simulink model "PMSM_mathmodel"  (R2018a)
settings: Solver=VariableStepAuto  StartTime=0.0  StopTime=2  RelTol=1e-3
libraries: nesl_utility x14, fl_lib x14, simulink x2, elec_lib x1
settings Model: Creator=Arpan  LastModifiedBy=Arpan

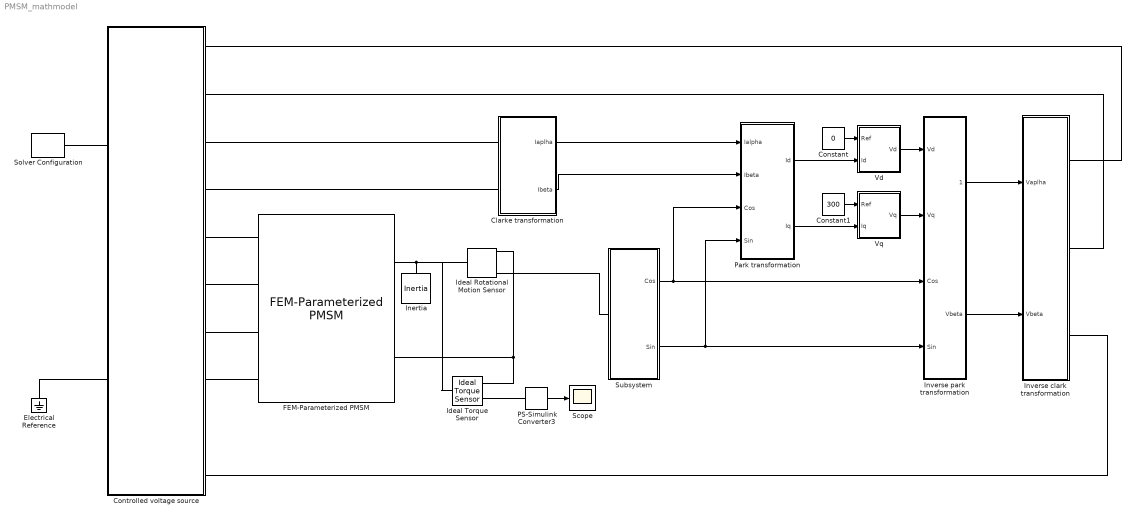
== system PMSM_mathmodel ==
  Clarke transformation : Subsystem
  Constant : Constant  Value=0
  Constant1 : Constant  Value=300
  Controlled voltage source : Subsystem
  Electrical Reference : fl_lib/Electrical/Electrical Elements/Electrical Reference
  FEM-Parameterized PMSM : elec_lib/Actuators & Drivers/Rotational Actuators/FEM-Parameterized PMSM  parameterization=2  iVec=[-2, 0, 2] A  xVec=[0, 20, 40, 60] deg  dfluxdiMatrix=0.0002 * ones(3, 4) Wb/A  dfluxdxMatrix=[0, -.16, .16, 0; 0, -.16, .16, 0; 0, -.16, .16, 0] Wb/rad  calculate_torque_matrix=1  TorqueMatrix=zeros(3, 3, 3, 4) N*m  idVec1=[-200, 0, 200] A  iqVec1=[-200, 0, 200] A  LdMatrix=0.0002 * ones(3, 3) H  LqMatrix=0.0002 * ones(3, 3) H  PmMatrix=0.1 * ones(3, 3) Wb  N=10  interp_method=simscape.enum.interpolation.linear  Rs=0.013 Ohm  Ms=0.00002 H  losses_oc=[0, 0, 0] W  losses_sc=[0, 0, 0] W  f_losses=60 Hz  Isc_losses=95 A  Inertia=0.1 kg*m^2  lam=0 N*m/(rad/s)  i_d_specify=on  i_d_priority=None  i_d=0.0085 A  i_d_nominal_specify=off  i_d_nominal_unit=A  i_d_nominal_value=1  i_q_specify=on  i_q_priority=None  i_q=0.0085 A  i_q_nominal_specify=off  i_q_nominal_unit=A  i_q_nominal_value=1  torque_specify=off  torque_priority=None  torque=0 N*m  torque_nominal_specify=off  torque_nominal_unit=N*m  torque_nominal_value=1  angular_velocity_specify=off  angular_velocity_priority=High  angular_velocity=0 rpm  angular_velocity_nominal_specify=off  angular_velocity_nominal_unit=rpm  angular_velocity_nominal_value=1  angular_position_specify=off  angular_position_priority=High  angular_position=0 deg  angular_position_nominal_specify=off  angular_position_nominal_unit=deg  angular_position_nominal_value=1  Tmeas=298.15 K  alpha=3.93e-3 1/K  alpha_flux=-0.001 1/K  stator_thermal_mass=100 J/K  stator_initial_temperatures=[298.15, 298.15, 298.15] K  rotor_thermal_mass=200 J/K  rotor_initial_temperature=298.15 K  Rm_percent_rotor=90  Rd_percent_rotor=30  idVec=[-200, 0, 200] A  iqVec=[-200, 0, 200] A  dfluxAdiaMatrix3D=zeros(3, 3, 4) Wb/A  dfluxAdibMatrix3D=zeros(3, 3, 4) Wb/A  dfluxAdicMatrix3D=zeros(3, 3, 4) Wb/A  dfluxAdxMatrix3D=zeros(3, 3, 4) Wb/rad  TorqueMatrix3D=zeros(3, 3, 4) N*m  iaVec=[-200, 0, 200] A  ibVec=[-200, 0, 200] A  icVec=[-200, 0, 200] A  dfluxAdiaMatrix=zeros(3, 3, 3, 4) Wb/A  dfluxAdibMatrix=zeros(3, 3, 3, 4) Wb/A  dfluxAdicMatrix=zeros(3, 3, 3, 4) Wb/A  dfluxAdxMatrix=zeros(3, 3, 3, 4) Wb/rad  winding_type_dq0=1  nPolePairs=4  parks_type=1  idVec2=[-200, 0, 200] A  iqVec2=[-200, 0, 200] A  xVec2=[0, 10, 20, 30] deg  fluxD_dq0=zeros(3, 3, 4) Wb  fluxQ_dq0=zeros(3, 3, 4) Wb  Torque_dq0=zeros(3, 3, 4) N*m
      settings: SourceProductName=Simscape Electronics  SourceProductBaseCode=SN
  Ideal Rotational Motion Sensor : fl_lib/Mechanical/Mechanical Sensors/Ideal Rotational Motion Sensor  offset=48 deg
  Ideal Torque Sensor : fl_lib/Mechanical/Mechanical Sensors/Ideal Torque Sensor
  Inertia : fl_lib/Mechanical/Rotational Elements/Inertia  inertia=0.01 kg*m^2  w_specify=off  w_priority=High  w=0 rad/s  w_nominal_specify=off  w_nominal_unit=rad/s  w_nominal_value=1  t_specify=off  t_priority=None  t=0 N*m  t_nominal_specify=off  t_nominal_unit=N*m  t_nominal_value=1
  Inverse clark transformation : Subsystem
  Inverse park transformation : Subsystem
  PS-Simulink Converter3 : nesl_utility/PS-Simulink Converter  PhysicalDomain=network_engine_domain  SubClassName=ps_output  LeftPortType=input  RightPortType=output  PseudoPeriodic=off  Frequencies=[]  Unit=1  AffineConversion=off
  Park transformation : Subsystem
  Scope : Scope
  Solver Configuration : nesl_utility/Solver Configuration  PhysicalDomain=network_engine_domain  SubClassName=solver  LeftPortType=input  RightPortType=generic  Tones=[]  Harmonics=[]  SimulateNoise=off  Profile=off  UseLocalSampling=off  EnableSwitchedLinearOptims=on  FrequencyDomain=off  UseCCode=off  RelTol=0.001  AbsTol=1e-06  MinStep=1e-09  ToWorkspace=off  RevertToSquareIcSolve=off  NumHomotopyIterations=100  PhasorMode=off  PhasorModeNumHarmonics=1  DoDC=off  ResidualTolerance=1e-09  UseLocalSolver=off  LocalSolverChoice=NE_BACKWARD_EULER_ADVANCER  LocalSolverSampleTime=0.001  DoFixedCost=off  MaxNonlinIter=3  MaxModeIter=2  LinearAlgebra=Sparse  EquationFormulation=NE_TIME_EF  DelaysMemoryBudget=1024  AutomaticFiltering=on  FilteringTimeConstant=0.001
  Subsystem : Subsystem
  Vd : Subsystem
  Vq : Subsystem
  wires:
  PS-Simulink Converter3/1 -> Scope/1
  Constant/1 -> Vd/1(Ref)
  Constant1/1 -> Vq/1(Ref)
  Clarke transformation/1(Iaplha) -> Park transformation/1(Ialpha)
  Clarke transformation/2(Ibeta) -> Park transformation/2(Ibeta)
  Park transformation/1(Id) -> Vd/2(Id)
  Park transformation/2(Iq) -> Vq/2(Iq)
  Vd/1(Vd) -> Inverse park transformation/1(Vd)
  Vq/1(Vq) -> Inverse park transformation/2(Vq)
  Inverse park transformation/1(Valpha) -> Inverse clark transformation/1(Vaplha)
  Inverse park transformation/2(Vbeta) -> Inverse clark transformation/2(Vbeta)
  Subsystem/1(Cos) -> Inverse park transformation/3(Cos), Park transformation/3(Cos)
  Subsystem/2(Sin) -> Inverse park transformation/4(Sin), Park transformation/4(Sin)
  connections:
  FEM-Parameterized PMSM/RConn1 -- Ideal Torque Sensor/LConn1 -- Ideal Rotational Motion Sensor/LConn1 -- Inertia/LConn1
  FEM-Parameterized PMSM/RConn2 -- Ideal Rotational Motion Sensor/RConn1 -- Ideal Torque Sensor/RConn1
  PS-Simulink Converter3/LConn1 -- Ideal Torque Sensor/RConn2
  Solver Configuration/RConn1 -- Controlled voltage source/LConn1
  Controlled voltage source/RConn3 -- Clarke transformation/LConn1
  Controlled voltage source/RConn4 -- Clarke transformation/LConn2
  Controlled voltage source/RConn5 -- FEM-Parameterized PMSM/LConn1
  Controlled voltage source/RConn6 -- FEM-Parameterized PMSM/LConn2
  Controlled voltage source/RConn7 -- FEM-Parameterized PMSM/LConn3
  Controlled voltage source/RConn8 -- FEM-Parameterized PMSM/LConn4
  Controlled voltage source/LConn2 -- Electrical Reference/LConn1
  Inverse clark transformation/RConn1 -- Controlled voltage source/RConn1
  Inverse clark transformation/RConn2 -- Controlled voltage source/RConn2
  Inverse clark transformation/RConn3 -- Controlled voltage source/RConn10
  Subsystem/LConn1 -- Ideal Rotational Motion Sensor/RConn3

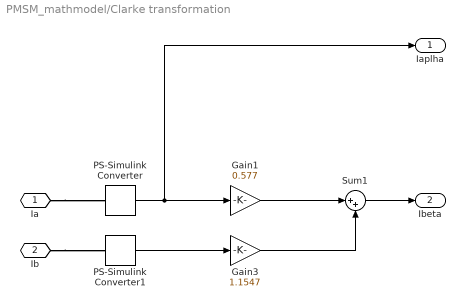
== system PMSM_mathmodel/Clarke transformation ==
  Gain1 : Gain  Gain=0.577
  Gain3 : Gain  Gain=1.1547
  PS-Simulink Converter : nesl_utility/PS-Simulink Converter  PhysicalDomain=network_engine_domain  SubClassName=ps_output  LeftPortType=input  RightPortType=output  PseudoPeriodic=off  Frequencies=[]  Unit=1  AffineConversion=off
  PS-Simulink Converter1 : nesl_utility/PS-Simulink Converter  PhysicalDomain=network_engine_domain  SubClassName=ps_output  LeftPortType=input  RightPortType=output  PseudoPeriodic=off  Frequencies=[]  Unit=1  AffineConversion=off
  Sum1 : Sum  Inputs=|++
  Ia : PMIOPort  Side=Left
  Ib : PMIOPort  Port=2  Side=Left
  Iaplha : Outport
  Ibeta : Outport  Port=2
  wires:
  Sum1/1 -> Ibeta/1
  Gain1/1 -> Sum1/1
  PS-Simulink Converter/1 -> Gain1/1, Iaplha/1
  Gain3/1 -> Sum1/2
  PS-Simulink Converter1/1 -> Gain3/1
  connections:
  Ib/RConn1 -- PS-Simulink Converter1/LConn1
  Ia/RConn1 -- PS-Simulink Converter/LConn1

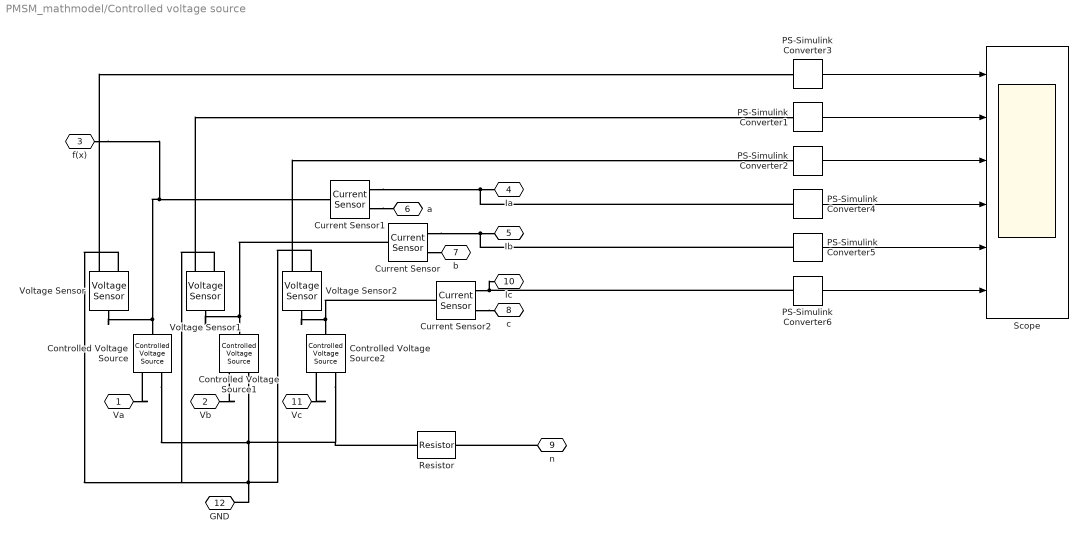
== system PMSM_mathmodel/Controlled voltage source ==
  Controlled Voltage Source : fl_lib/Electrical/Electrical Sources/Controlled Voltage Source
  Controlled Voltage Source1 : fl_lib/Electrical/Electrical Sources/Controlled Voltage Source
  Controlled Voltage Source2 : fl_lib/Electrical/Electrical Sources/Controlled Voltage Source
  Current Sensor : fl_lib/Electrical/Electrical Sensors/Current Sensor
  Current Sensor1 : fl_lib/Electrical/Electrical Sensors/Current Sensor
  Current Sensor2 : fl_lib/Electrical/Electrical Sensors/Current Sensor
  PS-Simulink Converter{1..6} (6 alike) : nesl_utility/PS-Simulink Converter  PhysicalDomain=network_engine_domain  SubClassName=ps_output  LeftPortType=input  RightPortType=output  PseudoPeriodic=off  Frequencies=[]  Unit=1  AffineConversion=off
  Resistor : fl_lib/Electrical/Electrical Elements/Resistor  R=1000 Ohm  i_specify=off  i_priority=None  i=0 A  i_nominal_specify=off  i_nominal_unit=A  i_nominal_value=1  v_specify=off  v_priority=None  v=0 V  v_nominal_specify=off  v_nominal_unit=V  v_nominal_value=1
  Scope : Scope  NumInputPorts=6
  Voltage Sensor : fl_lib/Electrical/Electrical Sensors/Voltage Sensor
  Voltage Sensor1 : fl_lib/Electrical/Electrical Sensors/Voltage Sensor
  Voltage Sensor2 : fl_lib/Electrical/Electrical Sensors/Voltage Sensor
  Va : PMIOPort  Side=Right
  Vb : PMIOPort  Port=2  Side=Right
  f(x) : PMIOPort  Port=3  Side=Left
  Ia : PMIOPort  Port=4  Side=Right
  Ib : PMIOPort  Port=5  Side=Right
  a : PMIOPort  Port=6  Side=Right
  b : PMIOPort  Port=7  Side=Right
  c : PMIOPort  Port=8  Side=Right
  n : PMIOPort  Port=9  Side=Right
  Ic : PMIOPort  Port=10  Side=Right
  Vc : PMIOPort  Port=11  Side=Right
  GND : PMIOPort  Port=12  Side=Left
  wires:
  PS-Simulink Converter3/1 -> Scope/1
  PS-Simulink Converter1/1 -> Scope/2
  PS-Simulink Converter2/1 -> Scope/3
  PS-Simulink Converter4/1 -> Scope/4
  PS-Simulink Converter5/1 -> Scope/5
  PS-Simulink Converter6/1 -> Scope/6
  connections:
  Current Sensor2/RConn1 -- Ic/RConn1 -- PS-Simulink Converter6/LConn1
  Current Sensor/RConn2 -- b/RConn1
  Current Sensor2/RConn2 -- c/RConn1
  Controlled Voltage Source/RConn2 -- Resistor/RConn1 -- Controlled Voltage Source2/RConn2 -- Voltage Sensor1/RConn2 -- Voltage Sensor/RConn2 -- Voltage Sensor2/RConn2 -- GND/RConn1 -- Controlled Voltage Source1/RConn2
  Current Sensor1/RConn1 -- PS-Simulink Converter4/LConn1 -- Ia/RConn1
  Current Sensor1/RConn2 -- a/RConn1
  Va/RConn1 -- Controlled Voltage Source/RConn1
  Vb/RConn1 -- Controlled Voltage Source1/RConn1
  Vc/RConn1 -- Controlled Voltage Source2/RConn1
  Current Sensor/RConn1 -- PS-Simulink Converter5/LConn1 -- Ib/RConn1
  f(x)/RConn1 -- Voltage Sensor/LConn1 -- Controlled Voltage Source/LConn1 -- Current Sensor1/LConn1
  Current Sensor/LConn1 -- Voltage Sensor1/LConn1 -- Controlled Voltage Source1/LConn1
  Current Sensor2/LConn1 -- Voltage Sensor2/LConn1 -- Controlled Voltage Source2/LConn1
  Voltage Sensor/RConn1 -- PS-Simulink Converter3/LConn1
  Voltage Sensor1/RConn1 -- PS-Simulink Converter1/LConn1
  Voltage Sensor2/RConn1 -- PS-Simulink Converter2/LConn1
  n/RConn1 -- Resistor/LConn1

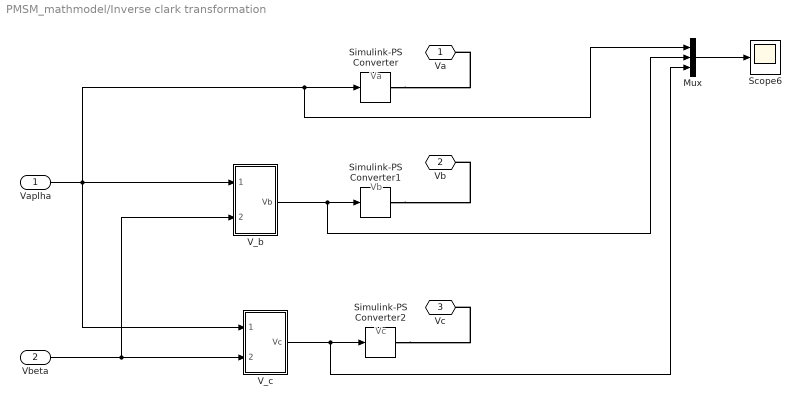
== system PMSM_mathmodel/Inverse clark transformation ==
  note: Vc
  note: Vb
  note: Va
  Vaplha : Inport
  Vbeta : Inport  Port=2
  Mux : Mux  Inputs=3
  Scope6 : Scope
  Simulink-PS Converter : nesl_utility/Simulink-PS Converter  PhysicalDomain=network_engine_domain  SubClassName=ps_input  LeftPortType=input  RightPortType=output  PseudoPeriodic=off  Frequencies=[]  NoiseDistribution=none  NoiseParameters=[]  Unit=1  AffineConversion=off  FilteringAndDerivatives=provide  SimscapeFilterOrder=1  InputFilterTimeConstant=0.001  UdotUserProvided=0
  Simulink-PS Converter1 : nesl_utility/Simulink-PS Converter  PhysicalDomain=network_engine_domain  SubClassName=ps_input  LeftPortType=input  RightPortType=output  PseudoPeriodic=off  Frequencies=[]  NoiseDistribution=none  NoiseParameters=[]  Unit=1  AffineConversion=off  FilteringAndDerivatives=provide  SimscapeFilterOrder=1  InputFilterTimeConstant=0.001  UdotUserProvided=0
  Simulink-PS Converter2 : nesl_utility/Simulink-PS Converter  PhysicalDomain=network_engine_domain  SubClassName=ps_input  LeftPortType=input  RightPortType=output  PseudoPeriodic=off  Frequencies=[]  NoiseDistribution=none  NoiseParameters=[]  Unit=1  AffineConversion=off  FilteringAndDerivatives=provide  SimscapeFilterOrder=1  InputFilterTimeConstant=0.001  UdotUserProvided=0
  V_b : Subsystem
  V_c : Subsystem
  Va : PMIOPort  Side=Right
  Vb : PMIOPort  Port=2  Side=Right
  Vc : PMIOPort  Port=3  Side=Right
  wires:
  Vbeta/1 -> V_c/2(Vbeta), V_b/2(Vbeta)
  Mux/1 -> Scope6/1
  V_c/1(Vc) -> Mux/3, Simulink-PS Converter2/1
  Vaplha/1 -> Mux/1, Simulink-PS Converter/1, V_b/1(Valpha), V_c/1(Valpha)
  V_b/1(Vb) -> Mux/2, Simulink-PS Converter1/1
  connections:
  Simulink-PS Converter1/RConn1 -- Vb/RConn1
  Simulink-PS Converter2/RConn1 -- Vc/RConn1
  Simulink-PS Converter/RConn1 -- Va/RConn1

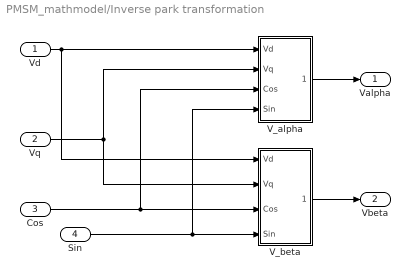
== system PMSM_mathmodel/Inverse park transformation ==
  Vd : Inport
  Vq : Inport  Port=2
  Cos : Inport  Port=3
  Sin : Inport  Port=4
  V_alpha : Subsystem
  V_beta : Subsystem
  Valpha : Outport
  Vbeta : Outport  Port=2
  wires:
  Sin/1 -> V_alpha/4(Sin), V_beta/4(Sin)
  Vd/1 -> V_alpha/1(Vd), V_beta/1(Vd)
  Cos/1 -> V_alpha/3(Cos), V_beta/3(Cos)
  V_beta/1(Vbeta) -> Vbeta/1
  V_alpha/1(Valpha) -> Valpha/1
  Vq/1 -> V_beta/2(Vq), V_alpha/2(Vq)

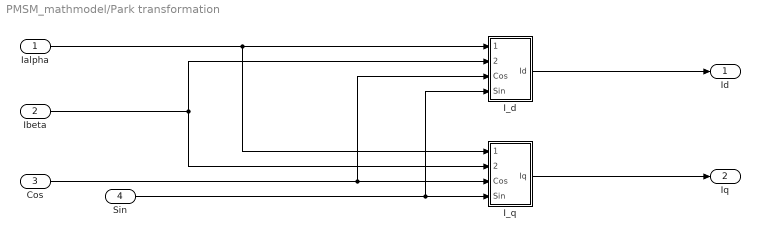
== system PMSM_mathmodel/Park transformation ==
  Ialpha : Inport
  Ibeta : Inport  Port=2
  Cos : Inport  Port=3
  Sin : Inport  Port=4
  I_d : Subsystem
  I_q : Subsystem
  Id : Outport
  Iq : Outport  Port=2
  wires:
  Cos/1 -> I_q/3(Cos), I_d/3(Cos)
  Ialpha/1 -> I_q/1(Ialpha), I_d/1(Iaplha)
  I_q/1(Iq) -> Iq/1
  Ibeta/1 -> I_q/2(Ibeta), I_d/2(Ibeta)
  Sin/1 -> I_d/4(Sin), I_q/4(Sin)
  I_d/1(Id) -> Id/1

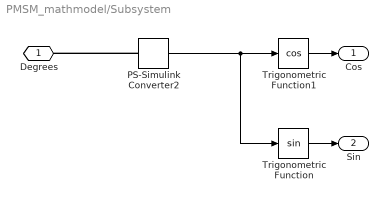
== system PMSM_mathmodel/Subsystem ==
  PS-Simulink Converter2 : nesl_utility/PS-Simulink Converter  PhysicalDomain=network_engine_domain  SubClassName=ps_output  LeftPortType=input  RightPortType=output  PseudoPeriodic=off  Frequencies=[]  Unit=1  AffineConversion=off
  Trigonometric Function : Trigonometry
  Trigonometric Function1 : Trigonometry  Operator=cos
  "Degrees " : PMIOPort  Side=Left
  Cos : Outport
  Sin : Outport  Port=2
  wires:
  PS-Simulink Converter2/1 -> Trigonometric Function/1, Trigonometric Function1/1
  Trigonometric Function1/1 -> Cos/1
  Trigonometric Function/1 -> Sin/1
  connections:
  PS-Simulink Converter2/LConn1 -- "Degrees "/RConn1

== system PMSM_mathmodel/Vd ==
  Ref : Inport
  Id : Inport  Port=2
  PID Controller (2DOF) : simulink/Continuous/PID Controller (2DOF)  Controller=PI  TimeDomain=Continuous-time  SampleTime=-1  IntegratorMethod=Forward Euler  FilterMethod=Forward Euler  Form=Parallel  UseFilter=on  ControllerParametersSource=internal  P=10  I=5  D=0  N=100  b=1  c=1  InitialConditionSource=internal  InitialConditionForIntegrator=0  InitialConditionForFilter=0  ExternalReset=none  LimitOutput=off  UpperSaturationLimit=inf  LowerSaturationLimit=-inf  LinearizeAsGain=on  AntiWindupMode=none  Kb=1  TrackingMode=off  Kt=1  PParamMin=[]  PParamMax=[]  IParamMin=[]  IParamMax=[]  DParamMin=[]  DParamMax=[]  NParamMin=[]  NParamMax=[]  bParamMin=[]  bParamMax=[]  cParamMin=[]  cParamMax=[]  KbParamMin=[]  KbParamMax=[]  KtParamMin=[]  KtParamMax=[]  POutMin=[]  POutMax=[]  IOutMin=[]  IOutMax=[]  DOutMin=[]  DOutMax=[]  NOutMin=[]  NOutMax=[]  bOutMin=[]  bOutMax=[]  cOutMin=[]  cOutMax=[]  KbOutMin=[]  KbOutMax=[]  KtOutMin=[]  KtOutMax=[]  IntegratorOutMin=[]  IntegratorOutMax=[]  FilterOutMin=[]  FilterOutMax=[]  SumOutMin=[]  SumOutMax=[]  Sum1OutMin=[]  Sum1OutMax=[]  Sum2OutMin=[]  Sum2OutMax=[]  Sum3OutMin=[]  Sum3OutMax=[]  SumI1OutMin=[]  SumI1OutMax=[]  SumI2OutMin=[]  SumI2OutMax=[]  SumI3OutMin=[]  SumI3OutMax=[]  SumDOutMin=[]  SumDOutMax=[]  SaturationOutMin=[]  SaturationOutMax=[]  IntegratorContinuousStateAttributes=''  IntegratorStateMustResolveToSignalObject=off  IntegratorRTWStateStorageClass=Auto  FilterContinuousStateAttributes=''  FilterStateMustResolveToSignalObject=off  FilterRTWStateStorageClass=Auto  DifferentiatorICPrevScaledInput=0  DifferentiatorOutMin=[]  DifferentiatorOutMax=[]  FilterDiffOutCoefMin=[]  FilterDiffOutCoefMax=[]  SumDenOutMin=[]  SumDenOutMax=[]  SumNumOutMin=[]  SumNumOutMax=[]  ReciprocalOutMin=[]  ReciprocalOutMax=[]  DivideOutMin=[]  DivideOutMax=[]  TunerSelectOption=Transfer Function Based (PID Tuner App)
  Vd : Outport
  wires:
  PID Controller (2DOF)/1 -> Vd/1
  Ref/1 -> PID Controller (2DOF)/1
  Id/1 -> PID Controller (2DOF)/2

== system PMSM_mathmodel/Vq ==
  Ref : Inport
  Iq : Inport  Port=2
  PID Controller (2DOF)1 : simulink/Continuous/PID Controller (2DOF)  Controller=PI  TimeDomain=Continuous-time  SampleTime=-1  IntegratorMethod=Forward Euler  FilterMethod=Forward Euler  Form=Parallel  UseFilter=on  ControllerParametersSource=internal  P=10  I=5  D=0  N=100  b=1  c=1  InitialConditionSource=internal  InitialConditionForIntegrator=0  InitialConditionForFilter=0  ExternalReset=none  LimitOutput=off  UpperSaturationLimit=inf  LowerSaturationLimit=-inf  LinearizeAsGain=on  AntiWindupMode=none  Kb=1  TrackingMode=off  Kt=1  PParamMin=[]  PParamMax=[]  IParamMin=[]  IParamMax=[]  DParamMin=[]  DParamMax=[]  NParamMin=[]  NParamMax=[]  bParamMin=[]  bParamMax=[]  cParamMin=[]  cParamMax=[]  KbParamMin=[]  KbParamMax=[]  KtParamMin=[]  KtParamMax=[]  POutMin=[]  POutMax=[]  IOutMin=[]  IOutMax=[]  DOutMin=[]  DOutMax=[]  NOutMin=[]  NOutMax=[]  bOutMin=[]  bOutMax=[]  cOutMin=[]  cOutMax=[]  KbOutMin=[]  KbOutMax=[]  KtOutMin=[]  KtOutMax=[]  IntegratorOutMin=[]  IntegratorOutMax=[]  FilterOutMin=[]  FilterOutMax=[]  SumOutMin=[]  SumOutMax=[]  Sum1OutMin=[]  Sum1OutMax=[]  Sum2OutMin=[]  Sum2OutMax=[]  Sum3OutMin=[]  Sum3OutMax=[]  SumI1OutMin=[]  SumI1OutMax=[]  SumI2OutMin=[]  SumI2OutMax=[]  SumI3OutMin=[]  SumI3OutMax=[]  SumDOutMin=[]  SumDOutMax=[]  SaturationOutMin=[]  SaturationOutMax=[]  IntegratorContinuousStateAttributes=''  IntegratorStateMustResolveToSignalObject=off  IntegratorRTWStateStorageClass=Auto  FilterContinuousStateAttributes=''  FilterStateMustResolveToSignalObject=off  FilterRTWStateStorageClass=Auto  DifferentiatorICPrevScaledInput=0  DifferentiatorOutMin=[]  DifferentiatorOutMax=[]  FilterDiffOutCoefMin=[]  FilterDiffOutCoefMax=[]  SumDenOutMin=[]  SumDenOutMax=[]  SumNumOutMin=[]  SumNumOutMax=[]  ReciprocalOutMin=[]  ReciprocalOutMax=[]  DivideOutMin=[]  DivideOutMax=[]  TunerSelectOption=Transfer Function Based (PID Tuner App)
  Vq : Outport
  wires:
  PID Controller (2DOF)1/1 -> Vq/1
  Ref/1 -> PID Controller (2DOF)1/1
  Iq/1 -> PID Controller (2DOF)1/2

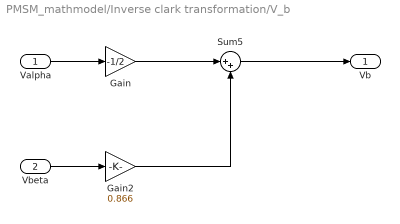
== system PMSM_mathmodel/Inverse clark transformation/V_b ==
  Valpha : Inport
  Vbeta : Inport  Port=2
  Gain : Gain  Gain=-1/2
  Gain2 : Gain  Gain=0.866
  Sum5 : Sum  Inputs=|++
  Vb : Outport
  wires:
  Gain/1 -> Sum5/1
  Gain2/1 -> Sum5/2
  Vbeta/1 -> Gain2/1
  Valpha/1 -> Gain/1
  Sum5/1 -> Vb/1

== system PMSM_mathmodel/Inverse clark transformation/V_c ==
  Valpha : Inport
  Vbeta : Inport  Port=2
  Gain4 : Gain  Gain=-1/2
  Gain5 : Gain  Gain=-0.866
  Sum6 : Sum  Inputs=|++
  Vc : Outport
  wires:
  Gain4/1 -> Sum6/1
  Valpha/1 -> Gain4/1
  Gain5/1 -> Sum6/2
  Vbeta/1 -> Gain5/1
  Sum6/1 -> Vc/1

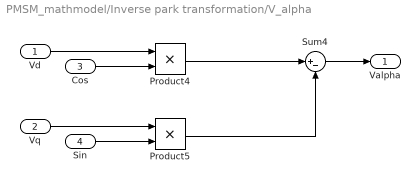
== system PMSM_mathmodel/Inverse park transformation/V_alpha ==
  Vd : Inport
  Vq : Inport  Port=2
  Cos : Inport  Port=3
  Sin : Inport  Port=4
  Product4 : Product
  Product5 : Product
  Sum4 : Sum  Inputs=|+-
  Valpha : Outport
  wires:
  Cos/1 -> Product4/2
  Product4/1 -> Sum4/1
  Product5/1 -> Sum4/2
  Sin/1 -> Product5/2
  Vd/1 -> Product4/1
  Sum4/1 -> Valpha/1
  Vq/1 -> Product5/1

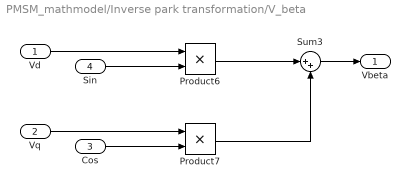
== system PMSM_mathmodel/Inverse park transformation/V_beta ==
  Vd : Inport
  Vq : Inport  Port=2
  Cos : Inport  Port=3
  Sin : Inport  Port=4
  Product6 : Product
  Product7 : Product
  Sum3 : Sum  Inputs=|++
  Vbeta : Outport
  wires:
  Product6/1 -> Sum3/1
  Vq/1 -> Product7/1
  Vd/1 -> Product6/1
  Product7/1 -> Sum3/2
  Cos/1 -> Product7/2
  Sum3/1 -> Vbeta/1
  Sin/1 -> Product6/2

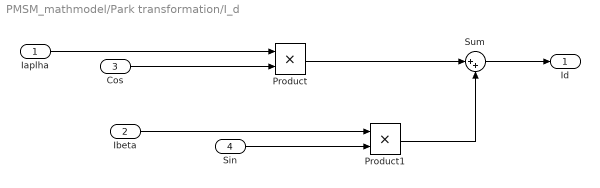
== system PMSM_mathmodel/Park transformation/I_d ==
  Iaplha : Inport
  Ibeta : Inport  Port=2
  Cos : Inport  Port=3
  Sin : Inport  Port=4
  Product : Product
  Product1 : Product
  Sum : Sum  Inputs=|++
  Id : Outport
  wires:
  Sin/1 -> Product1/2
  Product/1 -> Sum/1
  Product1/1 -> Sum/2
  Iaplha/1 -> Product/1
  Sum/1 -> Id/1
  Cos/1 -> Product/2
  Ibeta/1 -> Product1/1

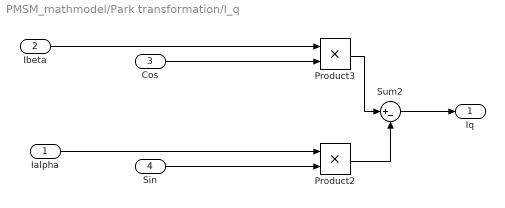
== system PMSM_mathmodel/Park transformation/I_q ==
  Ialpha : Inport
  Ibeta : Inport  Port=2
  Cos : Inport  Port=3
  Sin : Inport  Port=4
  Product2 : Product
  Product3 : Product
  Sum2 : Sum  Inputs=|+-
  Iq : Outport
  wires:
  Product3/1 -> Sum2/1
  Product2/1 -> Sum2/2
  Ialpha/1 -> Product2/1
  Sum2/1 -> Iq/1
  Sin/1 -> Product2/2
  Ibeta/1 -> Product3/1
  Cos/1 -> Product3/2
